simulink model "harmonic_analysis"  (R2016a)
settings: Solver=VariableStepAuto  StartTime=0.0  StopTime=Tfinal1  RelTol=1e-3
undefined symbols (not defined in the file): Ts, Ts1
libraries: powerlib x1
settings Model: Creator=mesutto  LastModifiedBy=mesutto

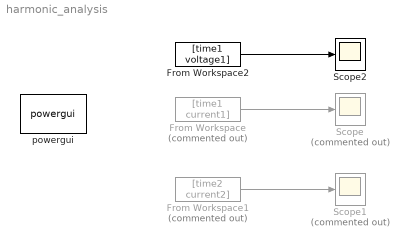
== system harmonic_analysis ==
  From Workspace : FromWorkspace  Commented=on  VariableName=[time1 current1]  OutDataTypeStr=double  SampleTime=Ts
  From Workspace1 : FromWorkspace  Commented=on  VariableName=[time2 current2]  OutDataTypeStr=double  SampleTime=Ts
  From Workspace2 : FromWorkspace  VariableName=[time1 voltage1]  OutDataTypeStr=double  SampleTime=Ts1
  Scope : Scope  Commented=on
  Scope1 : Scope  Commented=on
  Scope2 : Scope
  powergui : powerlib/powergui  Priority=1  SimulationMode=Discrete  SolverType=Tustin/Backward Euler (TBE)  SampleTime=Ts1  frequency=60  SPID=off  DisableSnubberDevices=off  DisableRonSwitches=off  DisableVfSwitches=off  SwTol=0  DisplayEquations=off  Interpol=off  ExternalGateDelay=off  methode=off  Ts=10  FunctionMessages=off  echomessages=off  HookPort=off  EnableUseOfTLC=off  x0status=blocks  frequencyindice=60  Pbase=100e6  ErrMax=1e-4  Iterations=50  UnitsV=kV  UnitsW=MW  buscounter=0  RestoreLinks=warning  ResistiveCurrentMeasurement=off  Frange=[0:2:500]  Ylog=off  Xlog=on  ShowGrid=off  save=off  variable=ZData  structure=ScopeData1  ZoomFFT=off  StartTime=0.0  cycles=2  DisplayStyle=1  fundamental=50  FreqAxis=off  MaxFrequency=50000  frequencyindicesteady=1  RmsSteady=1  display=off
  wires:
  From Workspace/1 -> Scope/1
  From Workspace1/1 -> Scope1/1
  From Workspace2/1 -> Scope2/1
